simulink model "modle"  (R2023a)
settings: Solver=VariableStepAuto  StartTime=0.0  StopTime=10  RelTol=1e-3
model workspace (MAT data in the model file):
  a = 0.05
(part 2 of 2)

== matlab function modle/Subsystem1/右后轮魔术轮胎Fx22/BCD ==
  data: Fz input; y output; b3 input; b4 input; b5 input
function y = fcn(Fz,b3,b4,b5)

y = (b3*Fz*Fz+b4*Fz)*exp(-b5*Fz);

== matlab function modle/MATLAB Function ==
  data: vx input; yawd output; deltaf input; mu input; betad output
function [yawd, betad]= fcn(vx,deltaf,mu)
m = 1412;
la = 1.015;
lb = 1.895;
L = la + lb;
Cf = -118610;
Cr = -94860;
g = 9.81;
% cr = -52000;
% cf = -34500;
g = 9.81;
K=m*(la/Cr-lb/Cf)/L^2;

YAWd1=vx*deltaf/L/(1+K*vx^2);
YAWd2 = 0.85*mu*g/vx;
yawd = min(abs(YAWd1),abs(YAWd2))*sign(YAWd1);

betad1=(la+m*lb*vx^2/L/Cr)*deltaf/((1+K*vx^2)*L);
betad2=mu*g*(lb/vx^2+m*la/Cr/L);
betad = min(abs(betad1),abs(betad2))*sign(betad1);

== matlab function modle/Subsystem1/MATLAB Function1 ==
  data: X input; miu12 output
function miu12 = get_slope(X)
    % 根据车辆位置X计算道路坡度cta
    % 输入:
    %   X - 车辆位置（米）
    % 输出:
    %   cta - 道路坡度

    if X >= 0 && X <= 30
        miu12 = 0.3;
    elseif X > 30 && X <= 60
        miu12 = 0.3;
    elseif X > 60 && X <= 100
        miu12 = 0.3;
    else
        error('X is out of the defined range (0 - 100 meters)');
    end
end

== matlab function modle/Subsystem1/右后轮魔术轮胎Fx22/D ==
  data: b1 input; y output; Fz input; b2 input
function y = fcn(b1,Fz,b2)

y = b1*Fz*Fz+b2*Fz+0.001;
